simulink model "PFFY"  (R2014b)
settings: Solver=ode45  StartTime=0.0  StopTime=10.0  RelTol=1e-3
libraries: dsparch4 x9, commnoisgen2 x1
settings Model: Creator=TY  LastModifiedBy=TY

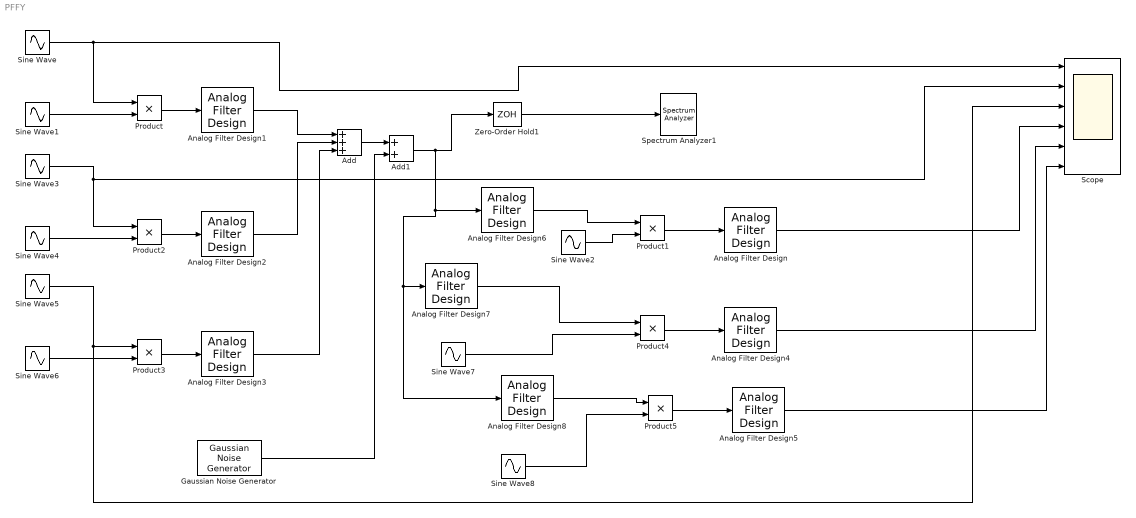
== system PFFY ==
  Add : Sum  Inputs=+++
  Add1 : Sum
  Analog Filter Design : dsparch4/Analog Filter Design  method=Butterworth  filttype=Lowpass  N=8  Wlo=15*6.28  Whi=80  Rp=2  Rs=40
  Analog Filter Design1 : dsparch4/Analog Filter Design  method=Butterworth  filttype=Bandpass  N=8  Wlo=185*6.28  Whi=195*6.28  Rp=2  Rs=40
  Analog Filter Design2 : dsparch4/Analog Filter Design  method=Butterworth  filttype=Bandpass  N=8  Wlo=275*6.28  Whi=285*6.28  Rp=2  Rs=40
  Analog Filter Design3 : dsparch4/Analog Filter Design  method=Butterworth  filttype=Bandpass  N=8  Wlo=365*6.28  Whi=375*6.28  Rp=2  Rs=40
  Analog Filter Design4 : dsparch4/Analog Filter Design  method=Butterworth  filttype=Lowpass  N=8  Wlo=25*6.28  Whi=80  Rp=2  Rs=40
  Analog Filter Design5 : dsparch4/Analog Filter Design  method=Butterworth  filttype=Lowpass  N=8  Wlo=35*6.28  Whi=80  Rp=2  Rs=40
  Analog Filter Design6 : dsparch4/Analog Filter Design  method=Butterworth  filttype=Bandpass  N=8  Wlo=185*6.28  Whi=195*6.28  Rp=2  Rs=40
  Analog Filter Design7 : dsparch4/Analog Filter Design  method=Butterworth  filttype=Bandpass  N=8  Wlo=275*6.28  Whi=285*6.28  Rp=2  Rs=40
  Analog Filter Design8 : dsparch4/Analog Filter Design  method=Butterworth  filttype=Bandpass  N=8  Wlo=365*6.28  Whi=375*6.28  Rp=2  Rs=40
  Gaussian Noise Generator : commnoisgen2/Gaussian Noise Generator  m=0  d=0  s=41  Ts=1/1000  frameBased=off  sampPerFrame=1  orient=off  outDataType=double
  Product{,1..5} (6 alike) : Product
  Scope : Scope  NumInputPorts=6
      settings: YMin=-5~-5~-5~-5~-5~-5  YMax=5~5~5~5~5~5
  Sine Wave : Sin  Frequency=10*6.28  SampleTime=0
  Sine Wave1 : Sin  Frequency=200*6.28  SampleTime=0
  Sine Wave2 : Sin  Frequency=200*6.28  SampleTime=0
  Sine Wave3 : Sin  Frequency=20*6.28  SampleTime=0
  Sine Wave4 : Sin  Frequency=300*6.28  SampleTime=0
  Sine Wave5 : Sin  Frequency=30*6.28  SampleTime=0
  Sine Wave6 : Sin  Frequency=400*6.28  SampleTime=0
  Sine Wave7 : Sin  Frequency=300*6.28  SampleTime=0
  Sine Wave8 : Sin  Frequency=400*6.28  SampleTime=0
  Spectrum Analyzer1 : SpectrumAnalyzer
  Zero-Order Hold1 : ZeroOrderHold  SampleTime=1/1000
  wires:
  Sine Wave/1 -> Product/1, Scope/1
  Sine Wave1/1 -> Product/2
  Sine Wave2/1 -> Product1/2
  Product1/1 -> Analog Filter Design/1
  Product/1 -> Analog Filter Design1/1
  Zero-Order Hold1/1 -> Spectrum Analyzer1/1
  Analog Filter Design1/1 -> Add/1
  Sine Wave3/1 -> Product2/1, Scope/2
  Sine Wave4/1 -> Product2/2
  Product2/1 -> Analog Filter Design2/1
  Sine Wave5/1 -> Scope/3, Product3/1
  Sine Wave6/1 -> Product3/2
  Product3/1 -> Analog Filter Design3/1
  Analog Filter Design2/1 -> Add/2
  Analog Filter Design3/1 -> Add/3
  Sine Wave7/1 -> Product4/2
  Product4/1 -> Analog Filter Design4/1
  Sine Wave8/1 -> Product5/2
  Product5/1 -> Analog Filter Design5/1
  Analog Filter Design6/1 -> Product1/1
  Analog Filter Design7/1 -> Product4/1
  Analog Filter Design8/1 -> Product5/1
  Add/1 -> Add1/1
  Gaussian Noise Generator/1 -> Add1/2
  Add1/1 -> Analog Filter Design8/1, Analog Filter Design7/1, Analog Filter Design6/1, Zero-Order Hold1/1
  Analog Filter Design/1 -> Scope/4
  Analog Filter Design4/1 -> Scope/5
  Analog Filter Design5/1 -> Scope/6
